simulink model "PianoPlayerSimulation"  (R2019b)
settings: Solver=VariableStepAuto  StartTime=0.0  StopTime=0  RelTol=1e-3
model workspace: external: MAT-File C:\Users\Alex\MATLAB Drive\PIANO PLAYER ARDUINO\OLDMC010.mat (data not in the file)
undefined symbols (not defined in the file or in its folder): A
settings Model: OrderedModelArguments=off  Creator=Alex  LastModifiedBy=Alex
settings DataIOCC: ExternalInput=[g]

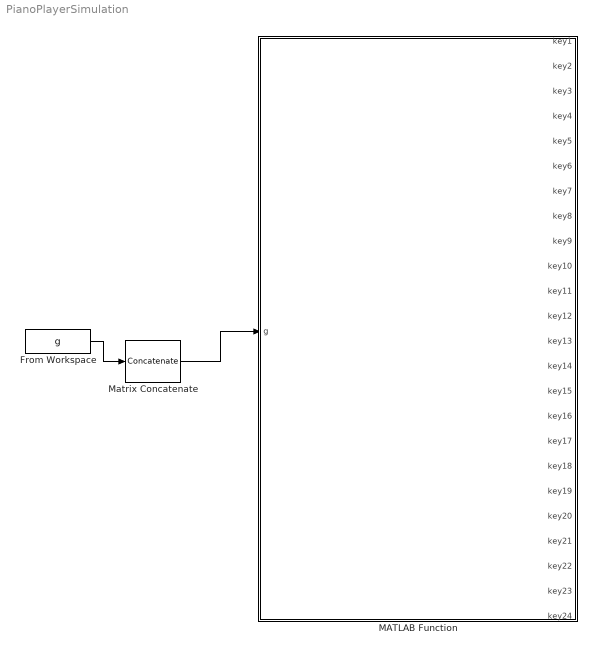
== system PianoPlayerSimulation ==
  From Workspace : FromWorkspace  VariableName=g  OutDataTypeStr=double  SampleTime=A  Interpolate=off  OutputAfterFinalValue=Setting to zero
  MATLAB Function : MATLAB Function  TreatAsAtomicUnit=on
  Matrix Concatenate : Concatenate  NumInputs=1  Mode=Multidimensional array  ConcatenateDimension=2
  wires:
  From Workspace/1 -> Matrix Concatenate/1
  Matrix Concatenate/1 -> MATLAB Function/1(g)

== matlab function PianoPlayerSimulation/MATLAB Function ==
  data: key1 output; key2 output; key3 output; key4 output; key5 output; key6 output; key7 output; key8 output; key9 output; key10 output; key11 output; key12 output; key13 output; key14 output; key15 output; key16 output; key17 output; key18 output; key19 output; key20 output; key21 output; key22 output; key23 output; key24 output; g input
function [key1,  key2,  key3,  key4,  key5,  key6,  key7,  key8,  key9,  key10,...
    key11, key12, key13, key14, key15, key16, key17, key18, key19, key20,...
    key21, key22, key23, key24]                              = STR2OUTPUT(g)


i = 1;

[r, c] = size(g);
while i < c + 1 %%ITERATE THROUGH EACH COLUMN
    j = 1;
    while j < r+1 %%TURN ON SPECIFIC PINS IN COLUMN
        if g(j,i) == 0 %%IF <missing> is value, end iteration.
            break
        else
            if g(j,i) == 22
                key1 = 1;
            elseif g(j,i) ==23
                key2 = 1;
                
            elseif g(j,i) ==24
                key3 = 1;
                
            elseif g(j,i) ==25
                key4 = 1;
                
            elseif g(j,i) ==26
                key5 = 1;
                
            elseif g(j,i) ==27
                key6 = 1;
                
            elseif g(j,i) ==28
                key7 = 1;
                
            elseif g(j,i) ==29
                key8 = 1;
                
            elseif g(j,i) ==30
                key9 = 1;
                
            elseif g(j,i) ==31
                key10 = 1;
                
            elseif g(j,i) ==32
                key11 = 1;
                
            elseif g(j,i) ==33
                key12 = 1;
                
            elseif g(j,i) ==34
                key13 = 1;
                
            elseif g(j,i) ==35
                key14 = 1;
                
            elseif g(j,i) ==36
                key15 = 1;
                
            elseif g(j,i) ==37
                key16 = 1;
                
            elseif g(j,i) ==38
                key17 = 1;
                
            elseif g(j,i) ==39
                key18 = 1;
                
            elseif g(j,i) ==40
                key19 = 1;
                
            elseif g(j,i) ==41
                key20 = 1;
                
            elseif g(j,i) ==42
                key21 = 1;
                
            elseif g(j,i) ==43
                key22 = 1;
                
            elseif g(j,i) ==44
                key23 = 1;
            elseif g(j,i) ==45
                key24 = 1;
                
            end
        end
        j = j+1;
    end
    pause(0.1); %%DELAY TO LET GO OF KEY BASED ON TIME MATRIX.
    j = 1;
    while j < r+1 %%TURN OFF SPECIFIC PINS IN COLUMN
        if g(j,i) == 0 %%IF <missing> is value, end iteration.
            break
        else
            if g(j,i) == 22
                key1 = 0;
            elseif g(j,i) ==23
                key2 = 0;
                
            elseif g(j,i) ==24
                key3 = 0;
                
            elseif g(j,i) ==25
                key4 = 0;
                
            elseif g(j,i) ==26
                key5 = 0;
                
            elseif g(j,i) ==27
                key6 = 0;
                
            elseif g(j,i) ==28
                key7 = 0;
                
            elseif g(j,i) ==29
                key8 = 0;
                
            elseif g(j,i) ==30
                key9 = 0;
                
            elseif g(j,i) ==31
                key10 =0;
                
            elseif g(j,i) ==32
                key11 = 0;
                
            elseif g(j,i) ==33
                key12 = 0;
                
            elseif g(j,i) ==34
                key13 = 0;
                
            elseif g(j,i) ==35
                key14 = 0;
                
            elseif g(j,i) ==36
                key15 = 0;
                
            elseif g(j,i) ==37
                key16 = 0;
                
            elseif g(j,i) ==38
                key17 = 0;
                
            elseif g(j,i) ==39
                key18 = 0;
                
            elseif g(j,i) ==40
                key19 = 0;
                
            elseif g(j,i) ==41
                key20 = 0;
                
            elseif g(j,i) ==42
                key21 = 0;
                
            elseif g(j,i) ==43
                key22 = 0;
                
            elseif g(j,i) ==44
                key23 = 0;
            elseif g(j,i) ==45
                key24 = 0;
                
            end
        end
        j = j+1;
    end
    i = i+1;
    pause(0.1); %%DELAY TO GO TO NEXT KEY BASED ON TIME MATRIX.
    %%GO TO NEXT COLUMN
    
end
end
